simulink model "model"  (R2020b)
settings: Solver=ode4  StartTime=0.0  StopTime=5.0  FixedStep=1/5000  RelTol=1e-3
settings Model: Creator=Pavan  LastModifiedBy=Pavan

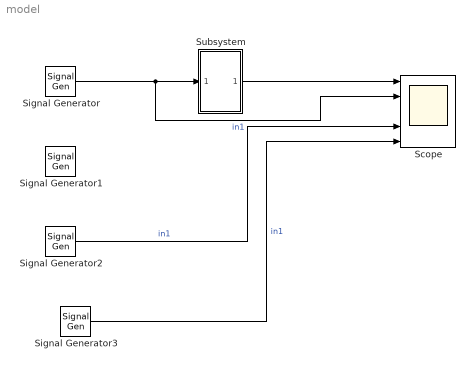
== system model ==
  Scope : Scope  NumInputPorts=5
  Signal Generator : SignalGenerator  Amplitude=5  Frequency=1000
  Signal Generator1 : SignalGenerator  Amplitude=5  Frequency=500
  Signal Generator2 : SignalGenerator  Amplitude=5  Frequency=1000
  Signal Generator3 : SignalGenerator  Amplitude=5  Frequency=4000
  Subsystem : Subsystem
  wires:
  Signal Generator/1 -> Scope/2, Subsystem/1(in1)  "in1"
  Signal Generator2/1 -> Scope/4  "in1"
  Signal Generator3/1 -> Scope/5  "in1"
  Subsystem/1(final) -> Scope/1

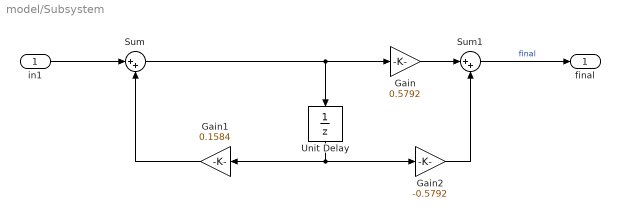
== system model/Subsystem ==
  in1 : Inport
  Gain : Gain  Gain=0.5792
  Gain1 : Gain  Gain=0.1584
  Gain2 : Gain  Gain=-0.5792
  Sum : Sum  Inputs=|++
  Sum1 : Sum  Inputs=|++
  Unit Delay : UnitDelay  SampleTime=-1  HasFrameUpgradeWarning=on
  final : Outport
  wires:
  in1/1 -> Sum/1
  Sum1/1 -> final/1  "final"
  Sum/1 -> Unit Delay/1, Gain/1
  Unit Delay/1 -> Gain2/1, Gain1/1
  Gain2/1 -> Sum1/2
  Gain1/1 -> Sum/2
  Gain/1 -> Sum1/1
